simulink model "AltitudeControllers"  (R2021a)
settings: Solver=VariableStepAuto  StartTime=0.0  StopTime=2500  FixedStep=0.0001  RelTol=1e-3
undefined symbols (not defined in the file): A_long, B_long, C_long, D_long, servo, theta0, U0, W0, X0
libraries: cstblocks x3, simulink_extras x2
settings Model: Creator=User01  LastModifiedBy=User01
settings SolverCC: ZeroCrossAlgorithm=Adaptive
settings DebuggingCC: IgnoredZcDiagnostic=none

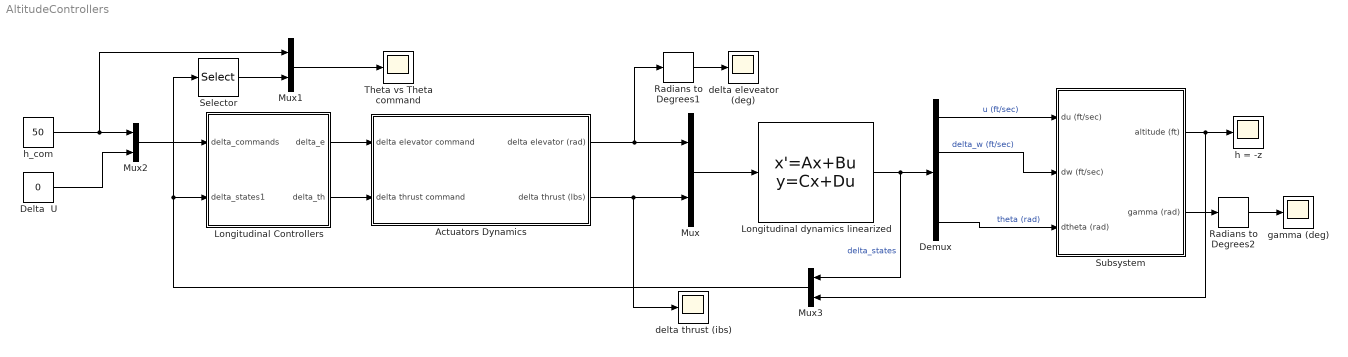
== system AltitudeControllers ==
  Actuators Dynamics : Subsystem
  Delta  U : Constant  Value=0
  Demux : Demux
  Longitudinal Controllers : Subsystem
  Longitudinal dynamics linearized : StateSpace  A=A_long  B=B_long  C=C_long  D=D_long  InitialCondition=0
  Mux{,1..3} (4 alike) : Mux  Inputs=2
  Radians to Degrees1 : simulink_extras/Transformations/Radians to Degrees
  Radians to Degrees2 : simulink_extras/Transformations/Radians to Degrees
  Selector : Selector  InputPortWidth=5  IndexOptions=Index vector (dialog)  Indices=5  OutputSizes=1
  Subsystem : Subsystem
  Theta vs Theta command : Scope
  delta eleveator (deg) : Scope
  delta thrust (ibs) : Scope
  gamma (deg) : Scope
  h = -z : Scope
  h_com : Constant  Value=50
  wires:
  Actuators Dynamics/2(delta thrust (lbs)) -> delta thrust (ibs)/1, Mux/2
  Mux2/1 -> Longitudinal Controllers/1(delta_commands)
  Delta  U/1 -> Mux2/2
  Demux/2 -> Subsystem/2(dw (ft/sec))  "delta_w (ft/sec)"
  Actuators Dynamics/1(delta elevator (rad)) -> Radians to Degrees1/1, Mux/1
  Longitudinal Controllers/1(delta_e) -> Actuators Dynamics/1(delta elevator command)
  Longitudinal Controllers/2(delta_th) -> Actuators Dynamics/2(delta thrust command)
  Mux/1 -> Longitudinal dynamics linearized/1
  Demux/4 -> Subsystem/3(dtheta (rad))  "theta (rad)"
  Mux1/1 -> Theta vs Theta command/1
  h_com/1 -> Mux2/1, Mux1/1
  Radians to Degrees2/1 -> gamma (deg)/1
  Demux/1 -> Subsystem/1(du (ft/sec))  "u (ft/sec)"
  Selector/1 -> Mux1/2
  Subsystem/1(altitude (ft)) -> Mux3/2, h = -z/1
  Longitudinal dynamics linearized/1 -> Mux3/1, Demux/1  "delta_states"
  Radians to Degrees1/1 -> delta eleveator (deg)/1
  Subsystem/2(gamma (rad)) -> Radians to Degrees2/1
  Mux3/1 -> Longitudinal Controllers/2(delta_states1), Selector/1

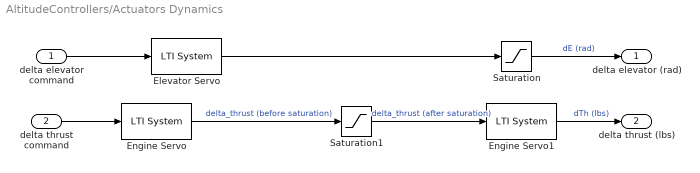
== system AltitudeControllers/Actuators Dynamics ==
  delta elevator command : Inport
  delta thrust command : Inport  Port=2
  Elevator Servo : cstblocks/LTI System  sys=-servo  IC=[]
  Engine Servo : cstblocks/LTI System  sys=servo  IC=[]
  Engine Servo1 : cstblocks/LTI System  sys=engine_timelag  IC=[]
  Saturation : Saturate  UpperLimit=25*pi/180  LowerLimit=-25*pi/180
  Saturation1 : Saturate  UpperLimit=47000  LowerLimit=-3*47000
  delta elevator (rad) : Outport
  delta thrust (lbs) : Outport  Port=2
  wires:
  Saturation/1 -> delta elevator (rad)/1  "dE (rad)"
  delta thrust command/1 -> Engine Servo/1
  Elevator Servo/1 -> Saturation/1
  Saturation1/1 -> Engine Servo1/1  "delta_thrust (after saturation)"
  Engine Servo/1 -> Saturation1/1  "delta_thrust (before saturation)"
  Engine Servo1/1 -> delta thrust (lbs)/1  "dTh (lbs)"
  delta elevator command/1 -> Elevator Servo/1

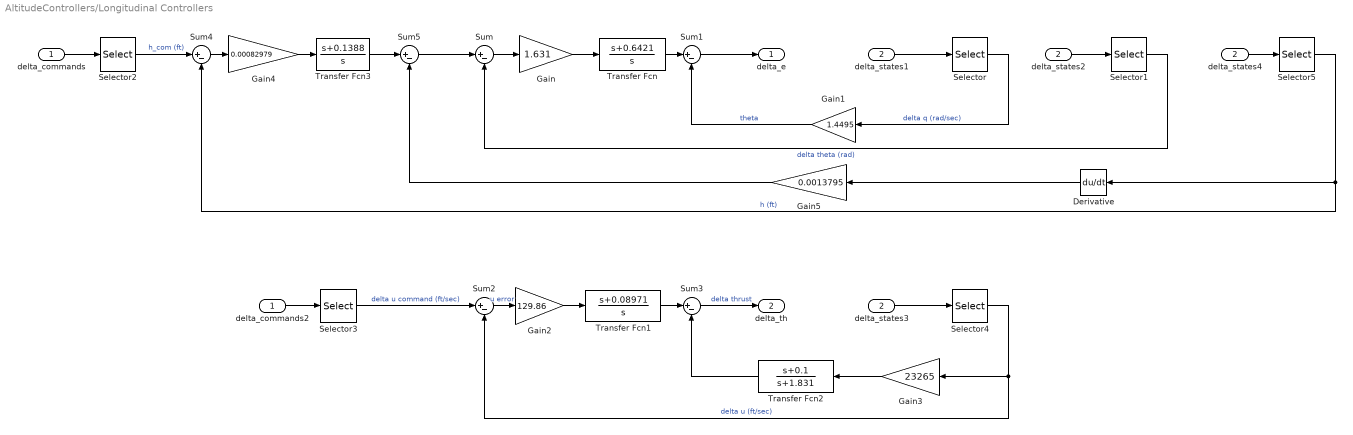
== system AltitudeControllers/Longitudinal Controllers ==
  delta_commands : Inport
  delta_states1 : Inport  Port=2
  Derivative : Derivative
  Gain : Gain  Gain=1.631
  Gain1 : Gain  Gain=1.4495
  Gain2 : Gain  Gain=129.86
  Gain3 : Gain  Gain=23265
  Gain4 : Gain  Gain=0.00082979
  Gain5 : Gain  Gain=0.0013795
  Selector : Selector  InputPortWidth=5  IndexOptions=Index vector (dialog)  Indices=3  OutputSizes=1
  Selector1 : Selector  InputPortWidth=5  IndexOptions=Index vector (dialog)  Indices=4  OutputSizes=1
  Selector2 : Selector  InputPortWidth=2  IndexOptions=Index vector (dialog)  Indices=1  OutputSizes=1
  Selector3 : Selector  InputPortWidth=2  IndexOptions=Index vector (dialog)  Indices=2  OutputSizes=1
  Selector4 : Selector  InputPortWidth=5  IndexOptions=Index vector (dialog)  Indices=1  OutputSizes=1
  Selector5 : Selector  InputPortWidth=5  IndexOptions=Index vector (dialog)  Indices=5  OutputSizes=1
  Sum{,1..5} (6 alike) : Sum  Inputs=|+-
  Transfer Fcn : TransferFcn  Numerator=[1 0.6421]  Denominator=[1 0]
  Transfer Fcn1 : TransferFcn  Numerator=[1 0.08971]  Denominator=[1 0]
  Transfer Fcn2 : TransferFcn  Numerator=[1 0.1]  Denominator=[1 1.831]
  Transfer Fcn3 : TransferFcn  Numerator=[1 0.1388]  Denominator=[1 0]
  delta_commands2 : InportShadow
  delta_states2 : InportShadow  Port=2
  delta_states3 : InportShadow  Port=2
  delta_states4 : InportShadow  Port=2
  delta_e : Outport
  delta_th : Outport  Port=2
  wires:
  Sum1/1 -> delta_e/1
  Transfer Fcn/1 -> Sum1/1
  Gain/1 -> Transfer Fcn/1
  Gain1/1 -> Sum1/2  "theta"
  Sum/1 -> Gain/1
  delta_commands/1 -> Selector2/1
  Selector2/1 -> Sum4/1  "h_com (ft)"
  delta_states1/1 -> Selector/1
  Selector/1 -> Gain1/1  "delta q (rad/sec)"
  delta_states2/1 -> Selector1/1
  Selector1/1 -> Sum/2  "delta theta (rad)"
  delta_commands2/1 -> Selector3/1
  delta_states3/1 -> Selector4/1
  Selector3/1 -> Sum2/1  "delta u command (ft/sec)"
  Selector4/1 -> Gain3/1, Sum2/2  "delta u (ft/sec)"
  Transfer Fcn1/1 -> Sum3/1
  Sum2/1 -> Gain2/1  "u error"
  Sum3/1 -> delta_th/1  "delta thrust"
  Transfer Fcn2/1 -> Sum3/2
  Gain2/1 -> Transfer Fcn1/1
  Gain3/1 -> Transfer Fcn2/1
  delta_states4/1 -> Selector5/1
  Selector5/1 -> Sum4/2, Derivative/1  "h (ft)"
  Transfer Fcn3/1 -> Sum5/1
  Sum5/1 -> Sum/1
  Gain4/1 -> Transfer Fcn3/1
  Sum4/1 -> Gain4/1
  Gain5/1 -> Sum5/2
  Derivative/1 -> Gain5/1

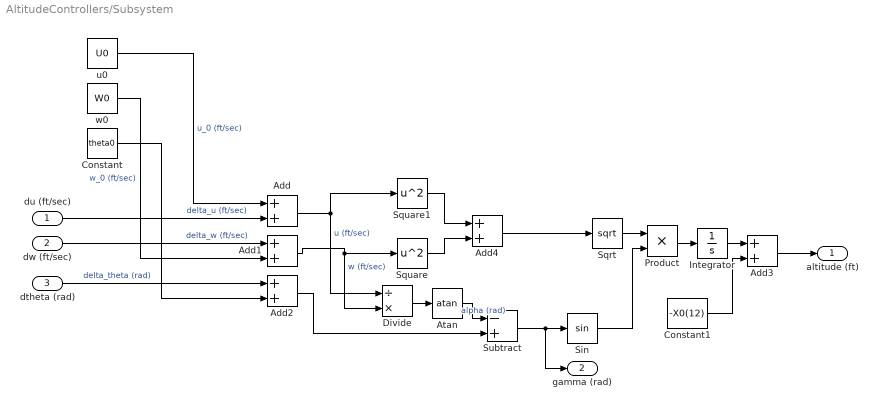
== system AltitudeControllers/Subsystem ==
  du (ft/sec) : Inport
  dw (ft/sec) : Inport  Port=2
  dtheta (rad) : Inport  Port=3
  Add{,1..4} (5 alike) : Sum
  Atan : Trigonometry  Operator=atan
  Constant : Constant  Value=theta0
  Constant1 : Constant  Value=-X0(12)
  Divide : Product  Inputs=/*
  Integrator : Integrator
  Product : Product
  Sin : Trigonometry
  Sqrt : Sqrt  SaturateOnIntegerOverflow=on
  Square : Math  Operator=square  SaturateOnIntegerOverflow=on
  Square1 : Math  Operator=square  SaturateOnIntegerOverflow=on
  Subtract : Sum  Inputs=-+
  u0 : Constant  Value=U0
  w0 : Constant  Value=W0
  altitude (ft) : Outport
  gamma (rad) : Outport  Port=2
  wires:
  Square/1 -> Add4/2
  Square1/1 -> Add4/1
  Add2/1 -> Subtract/2
  Sin/1 -> Product/2
  Add1/1 -> Divide/2, Square/1  "w (ft/sec)"
  Divide/1 -> Atan/1
  Sqrt/1 -> Product/1
  dw (ft/sec)/1 -> Add1/1  "delta_w (ft/sec)"
  Add3/1 -> altitude (ft)/1
  Atan/1 -> Subtract/1  "alpha (rad)"
  Constant1/1 -> Add3/2
  Add/1 -> Square1/1, Divide/1  "u (ft/sec)"
  du (ft/sec)/1 -> Add/2  "delta_u (ft/sec)"
  u0/1 -> Add/1  "u_0 (ft/sec)"
  Product/1 -> Integrator/1
  Add4/1 -> Sqrt/1
  w0/1 -> Add1/2  "w_0 (ft/sec)"
  dtheta (rad)/1 -> Add2/1  "delta_theta (rad)"
  Integrator/1 -> Add3/1
  Subtract/1 -> gamma (rad)/1, Sin/1
  Constant/1 -> Add2/2
